simulink model "mbed_SerialLoop"  (R2014a)
settings: Solver=FixedStepDiscrete  SolverMode=SingleTasking  StartTime=0.0  StopTime=10.0  FixedStep=1e-3  RelTol=1e-3
libraries: mbed_lib x3
settings Model: Creator=oh  LastModifiedBy=oh
settings OptimizationCC: OptimizeModelRefInitCode=on  LifeSpan=1
settings HardwareCC: ProdLargestAtomicInteger=Long  ProdLargestAtomicFloat=Double  ProdEndianess=LittleEndian  ProdHWDeviceType=ARM Compatible->ARM Cortex
settings RTWCC: SystemTargetFile=mbed.tlc  GenCodeOnly=on  TemplateMakefile=mbed.tmf  Description=Mbed Target (Embedded Target)  ProcessScript=mbed_make_rtw_hook  TargetLang=C++
settings CodeAppCC: IgnoreCustomStorageClasses=off
settings STFCustomTargetCC: TargetLibSuffix=.a  GenerateSampleERTMain=on  ConcurrentExecutionCompliant=off  GeneratePreprocessorConditionals=Use local settings  CombineOutputUpdateFcns=on  ERTCustomFileBanners=on  SupportContinuousTime=off  SupportNonInlinedSFcns=off  MATLABClassNameForMDSCustomization=Simulink.SoftwareTarget.ERTCustomization  GRTInterface=off  SystemTargetFile=mbed.tlc
settings ERTTargetCC: ERTCustomFileTemplate=mbed_file_process.tlc

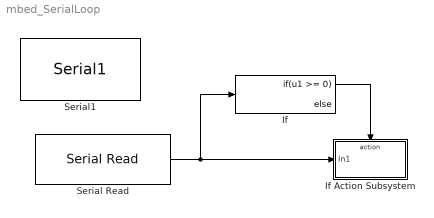
== system mbed_SerialLoop ==
  If : If  IfExpression=u1 >= 0
  If Action Subsystem : Subsystem  TreatAsAtomicUnit=on
  Serial Read : mbed_lib/Serial/Serial Read  SParameter1=Serial1  SampleTime=-1
  Serial1 : mbed_lib/DISCO_F407VG/Serial1  Parameter1=0
  wires:
  Serial Read/1 -> If Action Subsystem/1(In1), If/1
  If/1 -> If Action Subsystem/Action

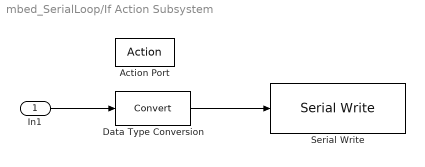
== system mbed_SerialLoop/If Action Subsystem ==
  In1 : Inport
  Action Port : ActionPort  ActionType=then
  Data Type Conversion : DataTypeConversion
  Serial Write : mbed_lib/Serial/Serial Write  SParameter1=Serial1  SampleTime=-1
  wires:
  Data Type Conversion/1 -> Serial Write/1
  In1/1 -> Data Type Conversion/1
